simulink model "rtwdemo_lct_start_term"  (Simulink 7.6)
settings: Solver=FixedStepDiscrete  StartTime=0.0  StopTime=20  FixedStep=0.01  RelTol=1e-3
libraries: rtwdemowidgets x2
Description:
  | Start and Terminate Actions
settings Model: Creator=The MathWorks Inc.  ExtModeAutoUpdateStatusClock=off
settings DataIOCC: SaveOutput=off  SaveTime=off  SignalLoggingName=sigsOut
settings OptimizationCC: InlineParams=on  InlineInvariantSignals=on  EfficientMapNaN2IntZero=off
settings DebuggingCC: SignalResolutionControl=TryResolveAllWithWarning  SolverPrmCheckMsg=none  MultiTaskDSMMsg=warning  MultiTaskCondExecSysMsg=none  StrictBusMsg=None
settings HardwareCC: TargetEndianess=LittleEndian  TargetHWDeviceType=MATLAB Host  ProdEqTarget=off
settings RTWCC: GenerateReport=on  RTWVerbose=off  ProcessScript=grt_make_rtw_hook  LaunchReport=on
settings GRTTargetCC: TargetFcnLib=ansi_tfl_tmw.mat

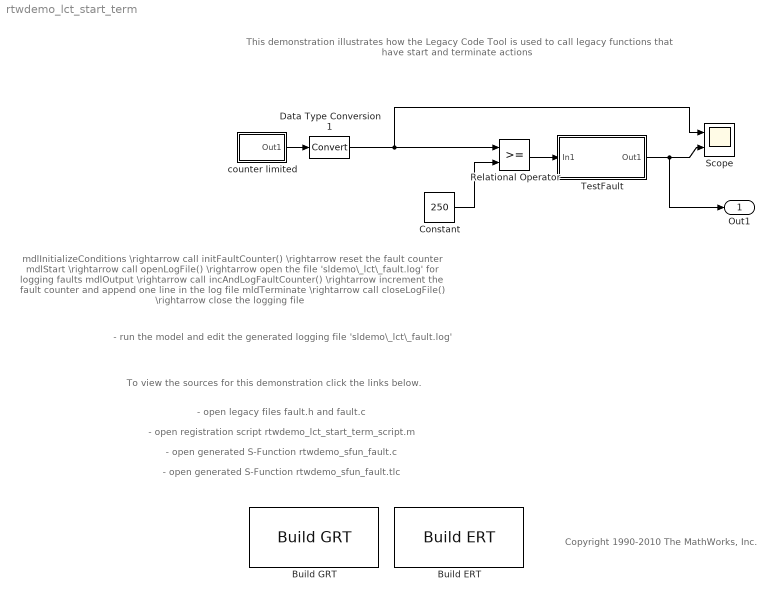
== system rtwdemo_lct_start_term ==
  note: Copyright 1990-2010 The MathWorks, Inc.
  note: This demonstration illustrates how the Legacy Code Tool is used to
      | call legacy functions that have start and terminate actions
  note: - open legacy files fault.h and fault.c
  note: To view the sources for this demonstration
      | click the links below.
  note: - open registration script rtwdemo_lct_start_term_script.m
  note: - open generated S-Function rtwdemo_sfun_fault.c
  note: - open generated S-Function rtwdemo_sfun_fault.tlc
  note: mdlInitializeConditions \rightarrow call initFaultCounter() \rightarrow reset the fault counter
      | mdlStart  \rightarrow call openLogFile()   \rightarrow open the file 'sldemo\_lct\_fault.log' for logging faults
      | mdlOutput \rightarrow call incAndLogFaultCounter()  \rightarrow increment the fault counter and append one line in the log file
      | mldTerminate  \rightarrow call closeLogFile()  \rightarrow close the logging file
  note: - run the model and edit the generated logging file 'sldemo\_lct\_fault.log'
  Build ERT : rtwdemowidgets/Build ERT  SystemSampleTime=-1  attrib_overrides={'IncludeMdlTerminateFcn'}
  Build GRT : rtwdemowidgets/Build GRT  SystemSampleTime=-1  attrib_overrides={}
  Constant : Constant  Value=250
  Data Type Conversion1 : DataTypeConversion  RndMeth=Zero
  Relational Operator : RelationalOperator  OutDataTypeStr=boolean
  Scope : Scope  NumInputPorts=2
      settings: TimeRange=20  YMin=0~0  YMax=300~50
  TestFault : Subsystem
  counter limited : Subsystem  mask(CounterLimited){th=2^8-1}
      mask prompts: th "Threshold:"
  Out1 : Outport
  wires:
  TestFault/1(Out1) -> Out1/1, Scope/2
  counter limited/1(Out1) -> Data Type Conversion1/1
  Data Type Conversion1/1 -> Scope/1, Relational Operator/1
  Relational Operator/1 -> TestFault/1(In1)
  Constant/1 -> Relational Operator/2

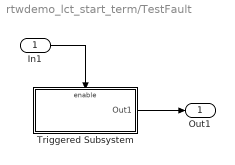
== system rtwdemo_lct_start_term/TestFault ==
  In1 : Inport
  Triggered Subsystem : Subsystem  TreatAsAtomicUnit=on
  Out1 : Outport
  wires:
  In1/1 -> Triggered Subsystem/Enable
  Triggered Subsystem/1(Out1) -> Out1/1

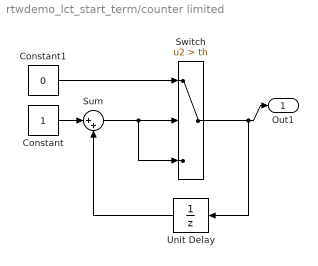
== system rtwdemo_lct_start_term/counter limited ==
  Constant : Constant
  Constant1 : Constant  Value=0
  Sum : Sum  Inputs=|++
  Switch : Switch  Criteria=u2 > Threshold  Threshold=th  ZeroCross=off
  Unit Delay : UnitDelay  X0=-1  SampleTime=-1
  Out1 : Outport
  wires:
  Constant/1 -> Sum/1
  Sum/1 -> Switch/2, Switch/3
  Unit Delay/1 -> Sum/2
  Constant1/1 -> Switch/1
  Switch/1 -> Unit Delay/1, Out1/1

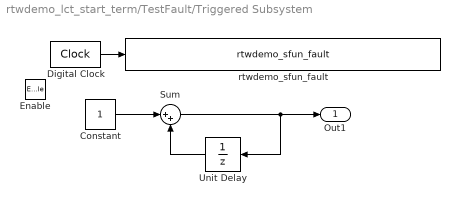
== system rtwdemo_lct_start_term/TestFault/Triggered Subsystem ==
  Enable : EnablePort
  Constant : Constant
  Digital Clock : DigitalClock  SampleTime=0.01
  Sum : Sum  Inputs=|++
  Unit Delay : UnitDelay  SampleTime=-1
  rtwdemo_sfun_fault : S-Function  FunctionName=rtwdemo_sfun_fault  EnableBusSupport=off  mask(Legacy Function){SFunctionSpec=incAndLogFaultCounter(void *work1, uint32 work2[1], double u1), ShowSpec=on}
      mask prompts: ShowSpec "Display function specification"
      mask help:
      | This block allows you to call the legacy functions specified by the following Legacy Code Tool definition:
      | def.SFunctionName = 'rtwdemo_sfun_fault';
      | def.InitializeConditionsFcnSpec = 'initFaultCounter(uint32 work2[1])';
      | def.OutputFcnSpec = 'incAndLogFaultCounter(void *work1, uint32 work2[1], double u1)';
      | def.StartFcnSpec = 'openLogFile(void **work1)';
      | def.TerminateFcnSpec = 'closeLogFile(void **work1)';
      | def.HeaderFiles = {'fault.h'};
      | def.SourceFiles = {'fault.c'};
      | def.IncPaths = {'sldemo_lct_src'};
      | def.SrcPaths = {'sldemo_lct_src'};
      | def.Options.useTlcWithAccel = false;
      mask Help: <p>This block was generated automatically by the Legacy Code Tool. For detailed help on this tool, call<a href="matlab:legacy_code('help')"> legacy_code('help')</a>.</p>
      mask CallbackString:
      | |if strcmp(get_param(gcbh, 'ShowSpec'), 'on')
      |   set_param(gcbh, 'MaskDisplay', sprintf('fprintf(''%s'');', get_param(gcbh, 'SFunctionSpec')));
      | else
      |   set_param(gcbh, 'MaskDisplay', sprintf('fprintf(''%s'');', get_param(gcbh, 'FunctionName')));
      | end
      mask Display: fprintf('incAndLogFaultCounter(void *work1, uint32 work2[1], double u1)');
  Out1 : Outport
  wires:
  Digital Clock/1 -> rtwdemo_sfun_fault/1
  Constant/1 -> Sum/1
  Sum/1 -> Unit Delay/1, Out1/1
  Unit Delay/1 -> Sum/2
